simulink model "SM24_model_W"  (R2025b)
settings: Solver=VariableStepAuto  StartTime=0.0  StopTime=T  MaxStep=1e-4  RelTol=1e-3  AbsTol=1e-6
InitFcn:
  | % =========================================================================
  | %  INIT CALLBACK — Simulink Model Workspace
  | %  Sistema de adquisición sísmica SM-24
  | % =========================================================================
  | 
  | %% ========================================================================
  | %  [ SECCIÓN 1: PARÁMETROS CONFIGURABLES ] (Editar solo aquí)
  | %  ========================================================================
  | 
  | % -------------------------------------------------------------------------
  | %  [1.1] Generales
  | % -------------------------------------------------------------------------
  | t_start  = 0;
  | 
  | % -------------------------------------------------------------------------
  | %  [1.2] Geófono SM-24
  | % -------------------------------------------------------------------------
  | fn  = 10;       % Frecuencia natural          (Hz)
  | hi  = 0.25;     % Amortiguamiento interno     (-)
  | G   = 28.8;     % Sensibilidad                (V·s/m)
  | m   = 0.011;    % Masa móvil                  (kg)
  | R_s = 375;      % Resistencia de bobina       (Ohm)
  | 
  | % -------------------------------------------------------------------------
  | %  [1.3] Etapa de Desacople
  | % -------------------------------------------------------------------------
  | R_d  = 1e6;     % Resistencia principal       (Ohm)
  | Ra_d = 10e3;    % Divisora A                  (Ohm)
  | Rb_d = 0;       % Divisora B                  (Ohm)
  | 
  | % -------------------------------------------------------------------------
  | %  [1.4] Diferencial a Single-Ended
  | % -------------------------------------------------------------------------
  | Ra_dse = 10e3;  % (Ohm)
  | Rb_dse = 220e3; % (Ohm)
  | 
  | % -------------------------------------------------------------------------
  | %  [1.5] Etapa de Acondicionamiento (Sallen-Key BP + Sumador)
  | % -------------------------------------------------------------------------
  | R1_bp        = 91000.0;   % (Ohm)
  | Rref_bp      = 82e3;   % (Ohm)
  | Ra_bp        = 22000.0;   % (Ohm)
  | Rb_bp        = 910000.0;  % (Ohm)
  | Rc_bp        = 8200.0;    % (Ohm)
  | C1_bp        = 0.00033;   % (F)
  | C2_bp        = 2.5e-12;   % (F)
  | 
  | Rin_bp_adder = 100000.0+60;  % (Ohm)
  | Rin_u_adder  = 2700.0;    % (Ohm)
  | Rf_add       = 270e3;   % (Ohm)
  | Cf_add       = 1.47e-9;     % (F)
  | Rref_add     = 2.7e3;    % (Ohm)
  | 
  | % -------------------------------------------------------------------------
  | %  [1.6] Filtro Anti-aliasing Analógico
  | % -------------------------------------------------------------------------
  | R1_aa = 270e3;    % (Ohm)
  | R2_aa = 39e3;     % (Ohm)
  | R3_aa = 18e3;     % (Ohm)
  | C1_aa = 33e-9;    % (F)
  | C2_aa = 820e-12;  % (F)
  | 
  | % -------------------------------------------------------------------------
  | %  [1.7] ADC Delta-Sigma
  | % -------------------------------------------------------------------------
  | Decimation_ADC = 64;     % Factor de decimación
  | Fs_ADC         = 3000;   % Frecuencia de muestreo de salida (Hz)
  | Vref           = 2.5;    % (V)
  | 
  | % -------------------------------------------------------------------------
  | %  [1.8] Filtro FIR (Parks-McClellan)
  | % -------------------------------------------------------------------------
  | N_fir = Fs_ADC/2;    % Orden del filtro
  | 
  | % -------------------------------------------------------------------------
  | %  [1.9] Señal de Excitación (3ra Derivada Gaussiana) — Multi-frecuencia
  | % -------------------------------------------------------------------------
  | f_g3_list  = [1];  % Frecuencias de los pulsos (Hz)
  | gap_cycles = 0.5;                          % Ciclos de silencio entre pulsos
  |                                          % (proporcional a cada frecuencia)
  | 
  | % -------------------------------------------------------------------------
  | %  [1.10] Ruido
  | % -------------------------------------------------------------------------
  | nivel_ruido      = 1;    % Ruido gaussiano (amplitud)
  | nivel_ruido_50Hz = 0.2;  % Interferencia de red (amplitud)
  | f_interferencia  = 50;   % Frecuencia de interferencia (Hz)
  | ruido_seed       = 42;   % Semilla fija (reproducibilidad + cache válido)
  | 
  | 
  | %% ========================================================================
  | %  [ SECCIÓN 2: CÁLCULOS Y VARIABLES DERIVADAS ] (No editar)
  | %  ========================================================================
  | 
  | % -------------------------------------------------------------------------
  | %  [2.1] Geófono — parámetros mecánicos y FT
  | % -------------------------------------------------------------------------
  | wn = 2 * pi * fn;
  | k  = m * wn^2;
  | d  = 2 * m * hi * wn;
  | 
  | N_geophone = [0,  wn,       0    ];
  | D_geophone = [1,  2*hi*wn,  wn^2 ];
  | 
  | % -------------------------------------------------------------------------
  | %  [2.2] Tiempos y frecuencias del ADC  (rápido, siempre calcular)
  | % -------------------------------------------------------------------------
  | Ts_ADC = 1 / (Fs_ADC * Decimation_ADC);   % Período modulador (s)
  | Nyq    = Fs_ADC / 2;                       % Frecuencia de Nyquist (Hz)
  | 
  | % -------------------------------------------------------------------------
  | %  [2.3 – 2.5] FIR + Señal + Ruido — con sistema de caché
  | % -------------------------------------------------------------------------
  | 
  | % Parámetros que determinan si el caché es válido
  | cache_file   = 'init_SM24_cache.mat';
  | cache_params = struct( ...
  |     'N_fir',            N_fir,            ...
  |     'Fs_ADC',           Fs_ADC,           ...
  |     'Decimation_ADC',   Decimation_ADC,   ...
  |     'f_g3_list',        f_g3_list,        ...
  |     'gap_cycles',       gap_cycles,       ...
  |     'nivel_ruido',      nivel_ruido,      ...
  |     'nivel_ruido_50Hz', nivel_ruido_50Hz, ...
  |     'f_interferencia',  f_interferencia,  ...
  |     'ruido_seed',       ruido_seed        ...
  | );
  | 
  | cache_valid = false;
  | if isfile(cache_file)
  |     try
  |         cached = load(cache_file);
  |         if isfield(cached, 'cache_params') && isequal(cached.cache_params, cache_params)
  |             cache_valid        = true;
  |             coeficientes_b     = cached.coeficientes_b;
  |             t                  = cached.t;
  |             g3                 = cached.g3;
  |             pulse_info         = cached.pulse_info;
  |             ruido              = cached.ruido;
  |             t_50Hz             = cached.t_50Hz;
  |             ruido_50Hz_diferencial = cached.ruido_50Hz_diferencial;
  |             T                  = cached.T;
  |             t_fir_delay        = cached.t_fir_delay;
  |             fprintf('[CACHE] Cargado desde "%s" — sin cambios detectados.\n', cache_file);
  |         else
  |             fprintf('[CACHE] Parámetros cambiaron — regenerando...\n');
  |         end
  |     catch
  |         fprintf('[CACHE] Archivo inválido — regenerando...\n');
  |     end
  | end
  | 
  | if ~cache_valid
  | 
  |     % -----------------------------------------------------------------------
  |     %  [2.3] Filtro FIR (Parks-McClellan)
  |     % -----------------------------------------------------------------------
  |     fprintf('[FIR] Calculando coeficientes (orden %d) — puede tardar...\n', N_fir);
  |     tic;
  |     coeficientes_b = firpm(N_fir, [0 130, 150 Nyq]/Nyq, [1 1, 0 0], ...
  |                            [1, 1/(10^(-100/20))]);
  |     fprintf('[FIR] Listo en %.1f s\n', toc);
  |     t_fir_delay = (N_fir * 0.75 + 5) / Fs_ADC;   % Latencia del FIR (s)
  | 
  |     % -----------------------------------------------------------------------
  |     %  [2.4] Señal multi-frecuencia (pulsos 3ra derivada gaussiana)
  |     % -----------------------------------------------------------------------
  | 
  |     % Pre-calcular duración de cada pulso y su gap de silencio
  |     sigmas = sqrt(3) ./ (2 * pi * f_g3_list);   % Ancho del pulso
  |     T_g3s  = 10 * sigmas;                        % Duración de cada pulso
  |     gaps   = gap_cycles ./ f_g3_list;            % Silencio proporcional
  | 
  |     % Tiempo total: todos los pulsos + gaps + latencia FIR
  |     T_senal = sum(T_g3s) + sum(gaps) + t_fir_delay;
  |     t       = 0 : Ts_ADC : T_senal;
  |     g3      = zeros(size(t));
  | 
  |     % Tabla de información de cada pulso (útil para análisis posterior)
  |     pulse_info = struct();
  |     pulse_info.freq       = f_g3_list;
  |     pulse_info.t_start    = zeros(size(f_g3_list));
  |     pulse_info.t_end      = zeros(size(f_g3_list));
  |     pulse_info.sigma      = sigmas;
  | 
  |     t_offset = 0;
  |     for k = 1 : numel(f_g3_list)
  |         sigma_k = sigmas(k);
  |         t0_k    = 5 * sigma_k;     % Centro del pulso dentro de su ventana
  |         T_g3_k  = T_g3s(k);
  |         gap_k   = gaps(k);
  | 
  |         t_start_k = t_offset;
  |         t_end_k   = t_offset + T_g3_k;
  | 
  |         % Índices del vector global que pertenecen a este pulso
  |         idx = (t >= t_start_k) & (t < t_end_k);
  | 
  |         % 3ra derivada gaussiana centrada en t0_k dentro de su ventana
  |         tau_k    = t(idx) - (t_start_k + t0_k);
  |         g3_k     = (tau_k .* (tau_k.^2 - 3*sigma_k^2) ./ sigma_k^6) ...
  |                    .* exp(-tau_k.^2 / (2*sigma_k^2));
  | 
  |         % Normalizar cada pulso individualmente a ±0.5
  |         pk = max(abs(g3_k));
  |         if pk > 0
  |             g3(idx) = g3_k / pk * 0.5;
  |         end
  | 
  |         pulse_info.t_start(k) = t_start_k;
  |         pulse_info.t_end(k)   = t_end_k;
  | 
  |         fprintf('[PULSO %d/%d] f=%.1f Hz | t=[%.3f, %.3f] s | sigma=%.4f s\n', ...
  |             k, numel(f_g3_list), f_g3_list(k), t_start_k, t_end_k, sigma_k);
  | 
  |         t_offset = t_end_k + gap_k;
  |     end
  | 
  |     % -----------------------------------------------------------------------
  |     %  [2.5] Generación de ruido (semilla fija para consistencia con caché)
  |     % -----------------------------------------------------------------------
  |     rng(ruido_seed);
  |     ruido = nivel_ruido * randn(size(g3));
  | 
  |     % Interferencia de red — un período completo
  |     t_50Hz                 = 0 : Ts_ADC : (1/f_interferencia - Ts_ADC);
  |     ruido_50Hz_diferencial = nivel_ruido_50Hz * sin(2*pi*f_interferencia*t_50Hz);
  | 
  |     % Duración total de simulación
  |     T = max(t(end), t_50Hz(end));
  | 
  |     % -----------------------------------------------------------------------
  |     %  Guardar caché
  |     % -----------------------------------------------------------------------
  |     save(cache_file, ...
  |         'cache_params', 'coeficientes_b', 't', 'g3', 'pulse_info', ...
  |         'ruido', 't_50Hz', 'ruido_50Hz_diferencial', 'T', 't_fir_delay');
  |     fprintf('[CACHE] Guardado en "%s"\n', cache_file);
  | 
  | end
  | set_param('SM24_model_W/Spectrum Analyzer', ...
  |     'FrequencySpan',  'Start and stop frequencies', ...
  |     'StartFrequency', num2str(min(f_g3_list) / 10), ...
  |     'StopFrequency',  num2str(Nyq));
  | fvtool(coeficientes_b, 1, 'Fs', Fs_ADC);
  | % -----------------------------------------------------------------------
  | %  Resumen final
  | % -----------------------------------------------------------------------
  | fprintf('\n--- Resumen de simulación ---\n');
  | fprintf('  Frecuencias:   %s Hz\n',  mat2str(f_g3_list));
  | fprintf('  T simulación:  %.2f s\n', T);
  | fprintf('  N muestras:    %.2fM\n',  numel(t)/1e6);
  | fprintf('  Ts_ADC:        %.2f µs\n', Ts_ADC*1e6);
  | fprintf('  Latencia FIR:  %.3f s\n', t_fir_delay);
  | fprintf('-----------------------------\n');
values from neighbouring files (symbols this model uses):
  s = tf('s')    [Compensador.m]    (also in compensadorKai.m)
libraries: fl_lib x55, nesl_utility x4, simulink x2, dspmlti4 x1, slctrl_linear x1
CloseFcn:
  | %% Script para unificar datos de Simulink en un solo archivo .mat
  | clear; clc; % <-- BORRAR o dejar comentado si se usa en el StopFcn de Simulink
settings Model: PacingRate=1000  Creator=elias  LastModifiedBy=elias
settings SolverCC: ZeroCrossAlgorithm=Adaptive
settings DebuggingCC: MaskedZcDiagnostic=none  IgnoredZcDiagnostic=none  ParameterPrecisionLossMsg=none
settings RTWCC: GPUComputeCapability=3.5

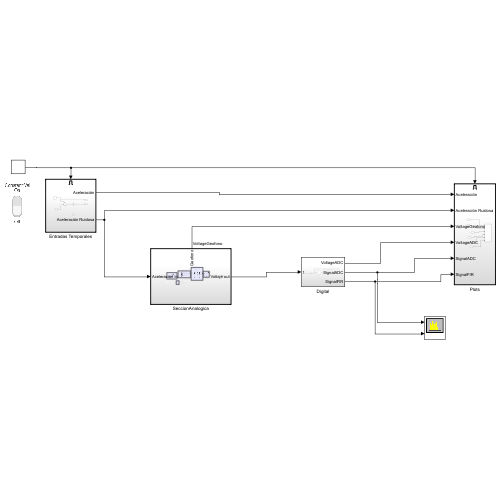
[thumbnail: Simulink's stored preview of the top-level diagram]
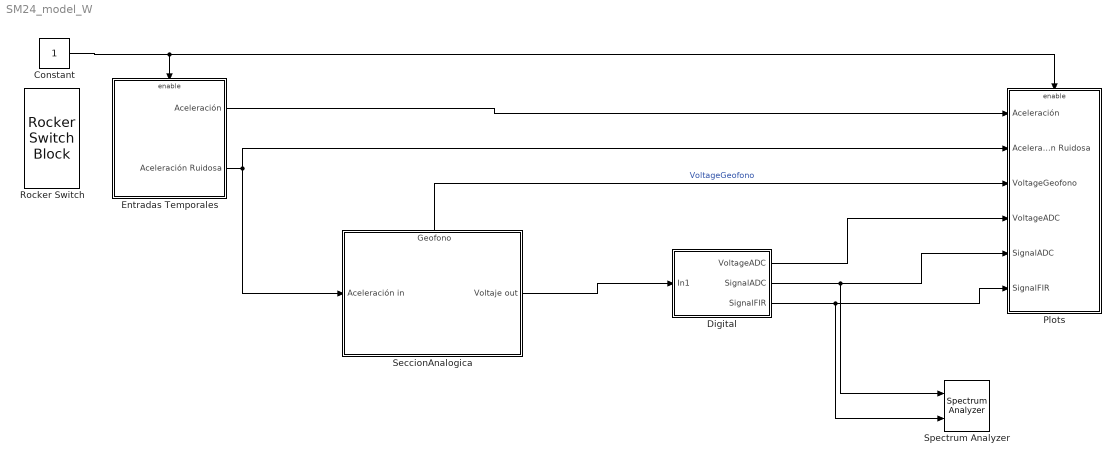
== system SM24_model_W ==
  Constant : Constant
  Digital : Subsystem
  Entradas Temporales : Subsystem
  Plots : Subsystem
  Rocker Switch : RockerSwitchBlock
  SeccionAnalogica : Subsystem  TreatAsAtomicUnit=on
      settings: PortSchema="{\"entries\":[{\"content\":{\"sides\":[{\"content\":{\"connectorIds\":[\"In1\"]},\"type\":\"ConnectorPlacement.EquallySpacedRectSide\",\"uuid\":\"1ba76ad7-8b54-4a44-9f91-ccc3badf3257\"},{\"content\":{\"connectorIds\":[\"Out1\"],\"side\":\"RIGHT\"},\"type\":\"ConnectorPlacement.EquallySpacedRectSide\",\"uuid\":\"9d848629-184e-471f-b904-52491969812c\"},{\"content\":{\"connectorIds\":[\"Out2\"],\"side\":\"TOP\"},\"type\":\"ConnectorPlacement.EquallySpacedRectSide\",\"uuid\":\"a82e2b6d-a8ff-4c30-87e4-e98957da3ec5\"},{\"content\":{\"side\":\"BOTTOM\"},\"type\":\"ConnectorPlacement.EquallySpacedRectSide\",\"uuid\":\"2899f004-1573-4205-9207-50e483759455\"}]},\"type\":\"ConnectorPlacement.EquallySpacedConnector\",\"uuid\":\"1d7f1859-f4c6-4ab5-a8c7-f48e1f148b97\"}],\"packageUris\":[\"http://schema.mathworks.com/mf0/Connector/R2020b\"],\"version\":\"1.0\"}"
  Spectrum Analyzer : SpectrumAnalyzer  NumInputPorts=2  WindowPosition=[481.000000,40.000000,958.000000,1000.000000,]  Visible=on  ScopeFrameLocation=window  ViewType=Spectrum and spectrogram  Method=Welch  SampleRate=44.1e3  PlotAsTwoSidedSpectrum=off  FrequencyScale=Log  WindowInvariantSamplesPerUpdate=on  FrequencySpan=Start and stop frequencies  StartFrequency=0.1  StopFrequency=1500  YLimits=[-3603.4449 -2802.6794]  ColorLimits=[-3603.4449 -2802.6794]  SelectedToolstripTab=spectrumAnalyzerToolstrip.spectrogramTab
  wires:
  SeccionAnalogica/2(Geofono) -> Plots/3(VoltageGeofono)  "VoltageGeofono"
  Constant/1 -> Plots/Enable, Entradas Temporales/Enable
  Entradas Temporales/1(Aceleración) -> Plots/1(Aceleración)
  Digital/3(SignalFIR) -> Spectrum Analyzer/2, Plots/6(SignalFIR)
  SeccionAnalogica/1(Voltaje out) -> Digital/1(In1)
  Digital/1(VoltageADC) -> Plots/4(VoltageADC)
  Digital/2(SignalADC) -> Spectrum Analyzer/1, Plots/5(SignalADC)
  Entradas Temporales/2(Aceleración Ruidosa) -> SeccionAnalogica/1(Aceleración in), Plots/2(Aceleración Ruidosa)

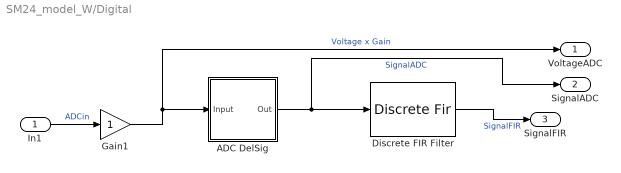
== system SM24_model_W/Digital ==
  In1 : Inport
  ADC DelSig : Subsystem
  Discrete FIR Filter : DiscreteFir  Coefficients=coeficientes_b
  Gain1 : Gain
  VoltageADC : Outport
  SignalADC : Outport  Port=2
  SignalFIR : Outport  Port=3
  wires:
  Discrete FIR Filter/1 -> SignalFIR/1  "SignalFIR"
  Gain1/1 -> VoltageADC/1, ADC DelSig/1(Input)  "Voltage x Gain"
  ADC DelSig/1(Out) -> SignalADC/1, Discrete FIR Filter/1  "SignalADC"
  In1/1 -> Gain1/1  "ADCin"

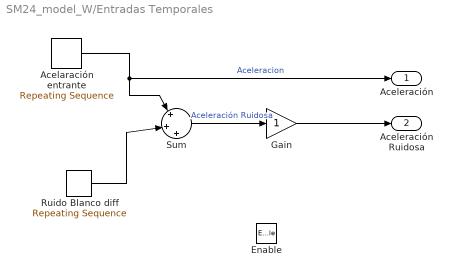
== system SM24_model_W/Entradas Temporales ==
  Enable : EnablePort
  Acelaración entrante : simulink/Sources/Repeating Sequence  rep_seq_t=t  rep_seq_y=g3
  Gain : Gain
  Ruido Blanco diff : simulink/Sources/Repeating Sequence  rep_seq_t=t  rep_seq_y=ruido
  Sum : Sum  Inputs=|+|+|+
  Aceleración : Outport
  Aceleración Ruidosa : Outport  Port=2
  wires:
  Acelaración entrante/1 -> Aceleración/1, Sum/1  "Aceleracion"
  Ruido Blanco diff/1 -> Sum/2
  Sum/1 -> Gain/1  "Aceleración Ruidosa"
  Gain/1 -> Aceleración Ruidosa/1

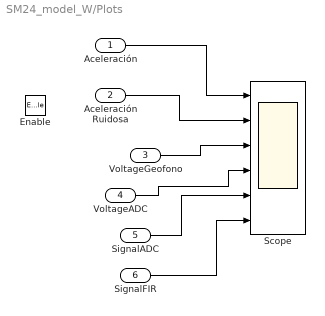
== system SM24_model_W/Plots ==
  Aceleración : Inport
  Aceleración Ruidosa : Inport  Port=2
  VoltageGeofono : Inport  Port=3
  VoltageADC : Inport  Port=4
  SignalADC : Inport  Port=5
  SignalFIR : Inport  Port=6
  Enable : EnablePort
  Scope : Scope  NumInputPorts=6
      settings: ActiveDisplayYMinimum=-89.67264371532174  ActiveDisplayYMaximum=50.94535948326461
  wires:
  Aceleración Ruidosa/1 -> Scope/2
  VoltageADC/1 -> Scope/4
  VoltageGeofono/1 -> Scope/3
  Aceleración/1 -> Scope/1
  SignalFIR/1 -> Scope/6
  SignalADC/1 -> Scope/5

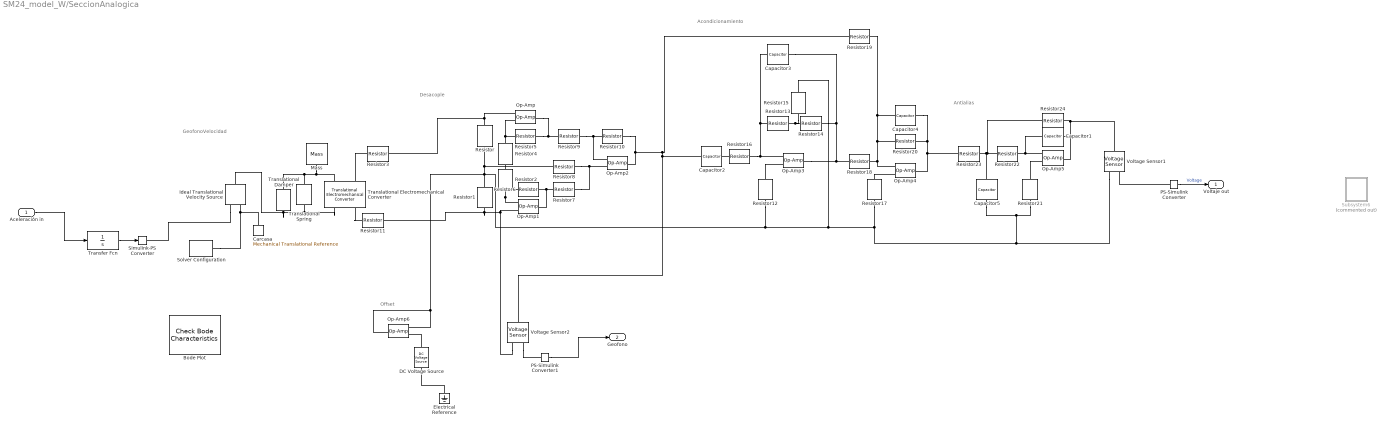
== system SM24_model_W/SeccionAnalogica ==
  note: Antialias
  note: Acondicionamiento
  note: GeofonoVelocidad
  note: Desacople
  note: Offset
  Aceleración in : Inport
  Bode Plot : slctrl_linear/Check Bode  Characteristics  InstantiateOnLoad=on  SaveOperatingPoints=off  LinearizationIOs={'/SeccionAnalogica/PS-Simulink Converter', 1, 'out', 'off', '';'/SeccionAnalogica/PS-Simulink Converter1', 1, 'out', 'off', '';'/SeccionAnalogica/Aceleración in', 1, 'in', 'off', ''}  LinearizeAt=SnapshotTimes  SnapshotTimes=[0]  TriggerType=rising  SampleTime=auto  RateConversionMethod=zoh  PreWarpFreq=10  UseExactDelayModel=off  UseFullBlockNameLabels=off  UseBusSignalLabels=off  enabled=on  stopWhenAssertionFail=off  export=off  ViewDlgPos=[2882 50 958 951]  OpenViewOnLoad=on  LaunchViewOnOpen=on  FrequencyUnits=rad/s  MagnitudeUnits=dB  PhaseUnits=deg  TimeUnits=seconds  EnableUpperBound=off  UpperBoundFrequencies=[]  UpperBoundMagnitudes=[]  EnableLowerBound=off  LowerBoundFrequencies=[]  LowerBoundMagnitudes=[]
      settings: LibrarySourceBlock=slctrlblks/Linear Analysis Plots/Bode Plot  SaveToWorkspace=off  SaveName=sys
  Capacitor1 : fl_lib/Electrical/Electrical Elements/Capacitor  c=C2_aa F  r=0 Ohm  g=0 1/Ohm  i_specify=off  i_priority=None  i=0 A  i_nominal_specify=off  i_nominal_value=1  i_nominal_unit=A  v_specify=off  v_priority=None  v=0 V  v_nominal_specify=off  v_nominal_value=1  v_nominal_unit=V  vc_specify=off  vc_priority=High  vc=0 V  vc_nominal_specify=off  vc_nominal_value=1  vc_nominal_unit=V
  Capacitor2 : fl_lib/Electrical/Electrical Elements/Capacitor  c=C1_bp F  r=0 Ohm  g=0 1/Ohm  i_specify=off  i_priority=None  i=0 A  i_nominal_specify=off  i_nominal_value=1  i_nominal_unit=A  v_specify=off  v_priority=None  v=0 V  v_nominal_specify=off  v_nominal_value=1  v_nominal_unit=V  vc_specify=off  vc_priority=High  vc=0 V  vc_nominal_specify=off  vc_nominal_value=1  vc_nominal_unit=V
  Capacitor3 : fl_lib/Electrical/Electrical Elements/Capacitor  c=C2_bp F  r=0 Ohm  g=0 1/Ohm  i_specify=off  i_priority=None  i=0 A  i_nominal_specify=off  i_nominal_value=1  i_nominal_unit=A  v_specify=off  v_priority=None  v=0 V  v_nominal_specify=off  v_nominal_value=1  v_nominal_unit=V  vc_specify=off  vc_priority=High  vc=0 V  vc_nominal_specify=off  vc_nominal_value=1  vc_nominal_unit=V
  Capacitor4 : fl_lib/Electrical/Electrical Elements/Capacitor  c=Cf_add F  r=0 Ohm  g=0 1/Ohm  i_specify=off  i_priority=None  i=0 A  i_nominal_specify=off  i_nominal_value=1  i_nominal_unit=A  v_specify=off  v_priority=None  v=0 V  v_nominal_specify=off  v_nominal_value=1  v_nominal_unit=V  vc_specify=off  vc_priority=High  vc=0 V  vc_nominal_specify=off  vc_nominal_value=1  vc_nominal_unit=V
  Capacitor5 : fl_lib/Electrical/Electrical Elements/Capacitor  c=C1_aa F  r=0 Ohm  g=0 1/Ohm  i_specify=off  i_priority=None  i=0 A  i_nominal_specify=off  i_nominal_value=1  i_nominal_unit=A  v_specify=off  v_priority=None  v=0 V  v_nominal_specify=off  v_nominal_value=1  v_nominal_unit=V  vc_specify=off  vc_priority=High  vc=0 V  vc_nominal_specify=off  vc_nominal_value=1  vc_nominal_unit=V
  Carcasa : fl_lib/Mechanical/Translational Elements/Mechanical Translational Reference
  DC Voltage Source : fl_lib/Electrical/Electrical Sources/DC Voltage Source  v0=2.5 V
  Electrical Reference : fl_lib/Electrical/Electrical Elements/Electrical Reference
  Ideal Translational Velocity Source : fl_lib/Mechanical/Mechanical Sources/Ideal Translational Velocity Source
  Mass : fl_lib/Mechanical/Translational Elements/Mass  mass=m kg  num_ports=foundation.enum.numPorts2.one  v_specify=off  v_priority=High  v=0 m/s  v_nominal_specify=off  v_nominal_value=1  v_nominal_unit=m/s  f_specify=off  f_priority=None  f=0 N  f_nominal_specify=off  f_nominal_value=1  f_nominal_unit=N
  Op-Amp{,1..6} (7 alike) : fl_lib/Electrical/Electrical Elements/Op-Amp  outI_specify=off  outI_priority=None  outI=0 A  outI_nominal_specify=off  outI_nominal_value=1  outI_nominal_unit=A
  PS-Simulink Converter : nesl_utility/PS-Simulink Converter  PhysicalDomain=network_engine_domain  SubClassName=ps_output  LeftPortType=input  RightPortType=output  PseudoPeriodic=off  Frequencies=[]  VectorFormat=inherit  Unit=inherit  AffineConversion=off
  PS-Simulink Converter1 : nesl_utility/PS-Simulink Converter  PhysicalDomain=network_engine_domain  SubClassName=ps_output  LeftPortType=input  RightPortType=output  PseudoPeriodic=off  Frequencies=[]  VectorFormat=inherit  Unit=inherit  AffineConversion=off
  Resistor : fl_lib/Electrical/Electrical Elements/Resistor  R=R_d Ohm  i_specify=off  i_priority=None  i=0 A  i_nominal_specify=off  i_nominal_value=1  i_nominal_unit=A  v_specify=off  v_priority=None  v=0 V  v_nominal_specify=off  v_nominal_value=1  v_nominal_unit=V
  Resistor1 : fl_lib/Electrical/Electrical Elements/Resistor  R=R_d Ohm  i_specify=off  i_priority=None  i=0 A  i_nominal_specify=off  i_nominal_value=1  i_nominal_unit=A  v_specify=off  v_priority=None  v=0 V  v_nominal_specify=off  v_nominal_value=1  v_nominal_unit=V
  Resistor10 : fl_lib/Electrical/Electrical Elements/Resistor  R=Rb_dse Ohm  i_specify=off  i_priority=None  i=0 A  i_nominal_specify=off  i_nominal_value=1  i_nominal_unit=A  v_specify=off  v_priority=None  v=0 V  v_nominal_specify=off  v_nominal_value=1  v_nominal_unit=V
  Resistor11 : fl_lib/Electrical/Electrical Elements/Resistor  R=R_s/2 Ohm  i_specify=off  i_priority=None  i=0 A  i_nominal_specify=off  i_nominal_value=1  i_nominal_unit=A  v_specify=off  v_priority=None  v=0 V  v_nominal_specify=off  v_nominal_value=1  v_nominal_unit=V
  Resistor12 : fl_lib/Electrical/Electrical Elements/Resistor  R=Rref_bp Ohm  i_specify=off  i_priority=None  i=0 A  i_nominal_specify=off  i_nominal_value=1  i_nominal_unit=A  v_specify=off  v_priority=None  v=0 V  v_nominal_specify=off  v_nominal_value=1  v_nominal_unit=V
  Resistor13 : fl_lib/Electrical/Electrical Elements/Resistor  R=Ra_bp Ohm  i_specify=off  i_priority=None  i=0 A  i_nominal_specify=off  i_nominal_value=1  i_nominal_unit=A  v_specify=off  v_priority=None  v=0 V  v_nominal_specify=off  v_nominal_value=1  v_nominal_unit=V
  Resistor14 : fl_lib/Electrical/Electrical Elements/Resistor  R=Rb_bp Ohm  i_specify=off  i_priority=None  i=0 A  i_nominal_specify=off  i_nominal_value=1  i_nominal_unit=A  v_specify=off  v_priority=None  v=0 V  v_nominal_specify=off  v_nominal_value=1  v_nominal_unit=V
  Resistor15 : fl_lib/Electrical/Electrical Elements/Resistor  R=Rc_bp Ohm  i_specify=off  i_priority=None  i=0 A  i_nominal_specify=off  i_nominal_value=1  i_nominal_unit=A  v_specify=off  v_priority=None  v=0 V  v_nominal_specify=off  v_nominal_value=1  v_nominal_unit=V
  Resistor16 : fl_lib/Electrical/Electrical Elements/Resistor  R=R1_bp Ohm  i_specify=off  i_priority=None  i=0 A  i_nominal_specify=off  i_nominal_value=1  i_nominal_unit=A  v_specify=off  v_priority=None  v=0 V  v_nominal_specify=off  v_nominal_value=1  v_nominal_unit=V
  Resistor17 : fl_lib/Electrical/Electrical Elements/Resistor  R=Rf_add Ohm  i_specify=off  i_priority=None  i=0 A  i_nominal_specify=off  i_nominal_value=1  i_nominal_unit=A  v_specify=off  v_priority=None  v=0 V  v_nominal_specify=off  v_nominal_value=1  v_nominal_unit=V
  Resistor18 : fl_lib/Electrical/Electrical Elements/Resistor  R=Rin_bp_adder Ohm  i_specify=off  i_priority=None  i=0 A  i_nominal_specify=off  i_nominal_value=1  i_nominal_unit=A  v_specify=off  v_priority=None  v=0 V  v_nominal_specify=off  v_nominal_value=1  v_nominal_unit=V
  Resistor19 : fl_lib/Electrical/Electrical Elements/Resistor  R=Rin_u_adder Ohm  i_specify=off  i_priority=None  i=0 A  i_nominal_specify=off  i_nominal_value=1  i_nominal_unit=A  v_specify=off  v_priority=None  v=0 V  v_nominal_specify=off  v_nominal_value=1  v_nominal_unit=V
  Resistor2 : fl_lib/Electrical/Electrical Elements/Resistor  R=Ra_d Ohm  i_specify=off  i_priority=None  i=0 A  i_nominal_specify=off  i_nominal_value=1  i_nominal_unit=A  v_specify=off  v_priority=None  v=0 V  v_nominal_specify=off  v_nominal_value=1  v_nominal_unit=V
  Resistor20 : fl_lib/Electrical/Electrical Elements/Resistor  R=Rf_add Ohm  i_specify=off  i_priority=None  i=0 A  i_nominal_specify=off  i_nominal_value=1  i_nominal_unit=A  v_specify=off  v_priority=None  v=0 V  v_nominal_specify=off  v_nominal_value=1  v_nominal_unit=V
  Resistor21 : fl_lib/Electrical/Electrical Elements/Resistor  R=Rf_add Ohm  i_specify=off  i_priority=None  i=0 A  i_nominal_specify=off  i_nominal_value=1  i_nominal_unit=A  v_specify=off  v_priority=None  v=0 V  v_nominal_specify=off  v_nominal_value=1  v_nominal_unit=V
  Resistor22 : fl_lib/Electrical/Electrical Elements/Resistor  R=R2_aa Ohm  i_specify=off  i_priority=None  i=0 A  i_nominal_specify=off  i_nominal_value=1  i_nominal_unit=A  v_specify=off  v_priority=None  v=0 V  v_nominal_specify=off  v_nominal_value=1  v_nominal_unit=V
  Resistor23 : fl_lib/Electrical/Electrical Elements/Resistor  R=R3_aa Ohm  i_specify=off  i_priority=None  i=0 A  i_nominal_specify=off  i_nominal_value=1  i_nominal_unit=A  v_specify=off  v_priority=None  v=0 V  v_nominal_specify=off  v_nominal_value=1  v_nominal_unit=V
  Resistor24 : fl_lib/Electrical/Electrical Elements/Resistor  R=R1_aa Ohm  i_specify=off  i_priority=None  i=0 A  i_nominal_specify=off  i_nominal_value=1  i_nominal_unit=A  v_specify=off  v_priority=None  v=0 V  v_nominal_specify=off  v_nominal_value=1  v_nominal_unit=V
  Resistor3 : fl_lib/Electrical/Electrical Elements/Resistor  R=R_s/2 Ohm  i_specify=off  i_priority=None  i=0 A  i_nominal_specify=off  i_nominal_value=1  i_nominal_unit=A  v_specify=off  v_priority=None  v=0 V  v_nominal_specify=off  v_nominal_value=1  v_nominal_unit=V
  Resistor4 : fl_lib/Electrical/Electrical Elements/Resistor  R=Ra_d Ohm  i_specify=off  i_priority=None  i=0 A  i_nominal_specify=off  i_nominal_value=1  i_nominal_unit=A  v_specify=off  v_priority=None  v=0 V  v_nominal_specify=off  v_nominal_value=1  v_nominal_unit=V
  Resistor5 : fl_lib/Electrical/Electrical Elements/Resistor  R=Rb_d Ohm  i_specify=off  i_priority=None  i=0 A  i_nominal_specify=off  i_nominal_value=1  i_nominal_unit=A  v_specify=off  v_priority=None  v=0 V  v_nominal_specify=off  v_nominal_value=1  v_nominal_unit=V
  Resistor6 : fl_lib/Electrical/Electrical Elements/Resistor  R=Rb_d Ohm  i_specify=off  i_priority=None  i=0 A  i_nominal_specify=off  i_nominal_value=1  i_nominal_unit=A  v_specify=off  v_priority=None  v=0 V  v_nominal_specify=off  v_nominal_value=1  v_nominal_unit=V
  Resistor7 : fl_lib/Electrical/Electrical Elements/Resistor  R=Ra_dse Ohm  i_specify=off  i_priority=None  i=0 A  i_nominal_specify=off  i_nominal_value=1  i_nominal_unit=A  v_specify=off  v_priority=None  v=0 V  v_nominal_specify=off  v_nominal_value=1  v_nominal_unit=V
  Resistor8 : fl_lib/Electrical/Electrical Elements/Resistor  R=Rb_dse Ohm  i_specify=off  i_priority=None  i=0 A  i_nominal_specify=off  i_nominal_value=1  i_nominal_unit=A  v_specify=off  v_priority=None  v=0 V  v_nominal_specify=off  v_nominal_value=1  v_nominal_unit=V
  Resistor9 : fl_lib/Electrical/Electrical Elements/Resistor  R=Ra_dse Ohm  i_specify=off  i_priority=None  i=0 A  i_nominal_specify=off  i_nominal_value=1  i_nominal_unit=A  v_specify=off  v_priority=None  v=0 V  v_nominal_specify=off  v_nominal_value=1  v_nominal_unit=V
  Simulink-PS Converter : nesl_utility/Simulink-PS Converter  PhysicalDomain=network_engine_domain  SubClassName=ps_input  LeftPortType=input  RightPortType=output  PseudoPeriodic=off  Frequencies=[]  NoiseDistribution=none  NoiseParameters=[]  Unit=1  AffineConversion=off  FilteringAndDerivatives=provide  SimscapeFilterOrder=1  InputFilterTimeConstant=0.001  UdotUserProvided=0
  Solver Configuration : nesl_utility/Solver Configuration  PhysicalDomain=network_engine_domain  SubClassName=solver  LeftPortType=input  RightPortType=generic  Tones=[]  Harmonics=[]  SimulateNoise=off  Profile=off  UseLocalSampling=off  EnableSwitchedLinearOptims=on  FrequencyDomain=off  UseCCode=off  RelTol=0.001  AbsTol=0.001  MinStep=1e-09  ToWorkspace=off  RevertToSquareIcSolve=off  NumHomotopyIterations=100  PhasorMode=off  PhasorModeNumHarmonics=1  ConsistencySolver=NEWTON_XTOL_AFTER_FTOL  IndexReductionMethod=DerivativeReplacement  DoDC=on  ResidualTolerance=1e-09  ConsistencyTolSource=GLOBAL  ConsistencyAbsTol=0.001  ConsistencyRelTol=0.001  ConsistencyTolFactor=0.001  UseLocalSolver=off  LocalSolverChoice=NE_BACKWARD_EULER_ADVANCER  ResolveIndetEquations=on  FunctionEvalNumThread=1  LocalSolverSampleTime=0.001  DoFixedCost=off  MaxNonlinIter=3  MaxModeIter=2  ComputeImpulses=off  ImpulseIterations=2  LinearAlgebra=auto  LinearAlgebraNumThread=0  EquationFormulation=NE_TIME_EF  DelaysMemoryBudget=1024  AutomaticFiltering=off  FilteringTimeConstant=0.001  PartitionStorageMethod=AS_NEEDED  PartitionMemoryBudget=1024  PartitionMethod=ROBUST  MultibodyUseLocalSolver=off  MultibodyLocalSolverChoice=ODE1  MultibodyLocalSolverSampleTime=0.001
  Subsystem6 : Subsystem  Commented=on
  Transfer Fcn : TransferFcn  Denominator=[1 0]
  Translational Electromechanical Converter : fl_lib/Electrical/Electrical Elements/Translational Electromechanical Converter  K=G V*s/m  i_specify=off  i_priority=None  i=0 A  i_nominal_specify=off  i_nominal_value=1  i_nominal_unit=A  v_specify=off  v_priority=None  v=0 V  v_nominal_specify=on  v_nominal_value=1  v_nominal_unit=V  f_specify=off  f_priority=None  f=0 N  f_nominal_specify=off  f_nominal_value=1  f_nominal_unit=N  u_specify=off  u_priority=None  u=0 m/s  u_nominal_specify=on  u_nominal_value=1  u_nominal_unit=m/s
      settings: InternalSimscapePortConfiguration="{\"Bottom\":[],\"Left\":[{\"id\":\"p\",\"label\":\"+\",\"type\":\"foundation.electrical.electrical\"},{\"id\":\"R\",\"label\":\"R\",\"type\":\"foundation.mechanical.translational.translational\"}],\"Right\":[{\"id\":\"n\",\"label\":\"-\",\"type\":\"foundation.electrical.electrical\"},{\"id\":\"C\",\"label\":\"C\",\"type\":\"foundation.mechanical.translational.translational\"}],\"Top\":[]}"
  Translational Damper : fl_lib/Mechanical/Translational Elements/Translational Damper  D=d N*s/m  v_specify=off  v_priority=None  v=0 m/s  v_nominal_specify=off  v_nominal_value=1  v_nominal_unit=m/s  f_specify=off  f_priority=None  f=0 N  f_nominal_specify=off  f_nominal_value=1  f_nominal_unit=N
  Translational Spring : fl_lib/Mechanical/Translational Elements/Translational Spring  spr_rate=k N/m  v_specify=off  v_priority=None  v=0 m/s  v_nominal_specify=off  v_nominal_value=1  v_nominal_unit=m/s  f_specify=off  f_priority=None  f=0 N  f_nominal_specify=off  f_nominal_value=1  f_nominal_unit=N  x_specify=off  x_priority=High  x=0 m  x_nominal_specify=off  x_nominal_value=1  x_nominal_unit=m
  Voltage Sensor1 : fl_lib/Electrical/Electrical Sensors/Voltage Sensor
  Voltage Sensor2 : fl_lib/Electrical/Electrical Sensors/Voltage Sensor
  Voltaje out : Outport
  Geofono : Outport  Port=2
  wires:
  PS-Simulink Converter1/1 -> Geofono/1
  Transfer Fcn/1 -> Simulink-PS Converter/1
  PS-Simulink Converter/1 -> Voltaje out/1  "Voltage"
  Aceleración in/1 -> Transfer Fcn/1
  connections:
  PS-Simulink Converter/LConn1 -- Voltage Sensor1/RConn1
  Resistor1/RConn1 -- Resistor15/RConn1 -- Capacitor5/RConn1 -- Resistor21/RConn1 -- Voltage Sensor1/RConn2 -- Resistor17/RConn1 -- Resistor12/RConn1 -- Op-Amp6/LConn1 -- Op-Amp6/RConn1 -- Resistor8/LConn1 -- Resistor/LConn1
  Ideal Translational Velocity Source/RConn1 -- Simulink-PS Converter/RConn1
  Resistor2/LConn1 -- Op-Amp1/LConn2 -- Resistor6/LConn1
  Electrical Reference/LConn1 -- DC Voltage Source/RConn1
  Resistor6/RConn1 -- Op-Amp1/RConn1 -- Resistor7/LConn1
  Translational Electromechanical Converter/LConn1 -- Resistor3/LConn1
  Resistor5/RConn1 -- Op-Amp/RConn1 -- Resistor9/LConn1
  Translational Damper/RConn1 -- Ideal Translational Velocity Source/LConn1 -- Translational Electromechanical Converter/RConn2 -- Translational Spring/RConn1
  Resistor4/RConn1 -- Op-Amp/LConn2 -- Resistor5/LConn1
  Translational Spring/LConn1 -- Translational Electromechanical Converter/LConn2 -- Mass/LConn1 -- Translational Damper/LConn1
  DC Voltage Source/LConn1 -- Op-Amp6/LConn2
  Carcasa/LConn1 -- Solver Configuration/RConn1 -- Ideal Translational Velocity Source/RConn2
  Resistor1/LConn1 -- Op-Amp1/LConn1 -- Voltage Sensor2/RConn2 -- Resistor11/RConn1
  Voltage Sensor2/RConn1 -- PS-Simulink Converter1/LConn1
  Resistor7/RConn1 -- Op-Amp2/LConn1 -- Resistor8/RConn1
  Resistor9/RConn1 -- Resistor10/LConn1 -- Op-Amp2/LConn2
  Resistor2/RConn1 -- Resistor4/LConn1
  Resistor11/LConn1 -- Translational Electromechanical Converter/RConn1
  Resistor/RConn1 -- Op-Amp/LConn1 -- Resistor3/RConn1
  Resistor12/LConn1 -- Op-Amp3/LConn1
  Capacitor3/LConn1 -- Op-Amp3/LConn2 -- Resistor16/LConn1 -- Resistor13/RConn1
  Resistor10/RConn1 -- Voltage Sensor2/LConn1 -- Capacitor2/LConn1 -- Resistor19/LConn1 -- Op-Amp2/RConn1
  Op-Amp4/LConn1 -- Resistor17/LConn1
  Resistor18/RConn1 -- Op-Amp4/LConn2 -- Resistor19/RConn1 -- Capacitor4/LConn1 -- Resistor20/LConn1
  Capacitor4/RConn1 -- Resistor23/LConn1 -- Op-Amp4/RConn1 -- Resistor20/RConn1
  Resistor21/LConn1 -- Op-Amp5/LConn1
  Resistor22/RConn1 -- Op-Amp5/LConn2 -- Capacitor1/LConn1
  Capacitor1/RConn1 -- Voltage Sensor1/LConn1 -- Resistor24/RConn1 -- Op-Amp5/RConn1
  Resistor23/RConn1 -- Resistor22/LConn1 -- Resistor24/LConn1 -- Capacitor5/LConn1
  Resistor18/LConn1 -- Capacitor3/RConn1 -- Resistor14/LConn1 -- Op-Amp3/RConn1
  Capacitor2/RConn1 -- Resistor16/RConn1
  Resistor15/LConn1 -- Resistor13/LConn1 -- Resistor14/RConn1

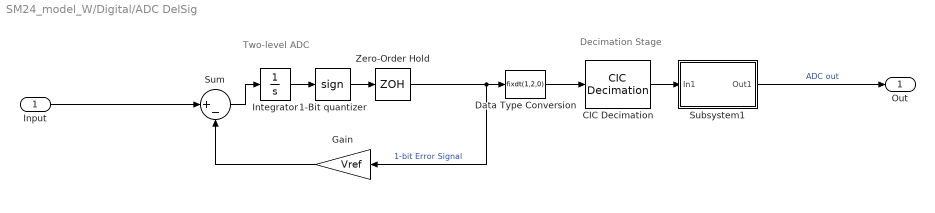
== system SM24_model_W/Digital/ADC DelSig ==
  note: Two-level ADC
  note: Decimation Stage
  Input : Inport
  1-Bit quantizer : Signum
  CIC Decimation : dspmlti4/CIC Decimation  filtFrom=Dialog parameters  filtobj=Hm_decim  ftype=Decimator  R=Decimation_ADC  M=1  N=5  filterInternals=Full precision  BPS=[32 30 24 20 16 16 16 16 16 16]  FLPS=0  outputWordLength=16  outputFracLength=0  launchFVT=off  framing=Maintain input frame rate  RateOptions=Allow multirate processing
  Data Type Conversion : DataTypeConversion  OutDataTypeStr=fixdt(1,2,0)  SaturateOnIntegerOverflow=off  RndMeth=Floor
  Gain : Gain  Gain=Vref
  Integrator : Integrator
  Subsystem1 : Subsystem
      mask Display: disp('Rescaling for\nComparison')
  Sum : Sum  Inputs=|+-  InputSameDT=on  SaturateOnIntegerOverflow=on  OutDataTypeStr=Inherit: Same as first input
  Zero-Order Hold : ZeroOrderHold  SampleTime=Ts_ADC
  Out : Outport
  wires:
  Data Type Conversion/1 -> CIC Decimation/1
  Zero-Order Hold/1 -> Gain/1, Data Type Conversion/1  "1-bit Error Signal"
  Integrator/1 -> 1-Bit quantizer/1
  1-Bit quantizer/1 -> Zero-Order Hold/1
  Sum/1 -> Integrator/1
  Input/1 -> Sum/1
  CIC Decimation/1 -> Subsystem1/1(In1)
  Subsystem1/1(Out1) -> Out/1  "ADC out"
  Gain/1 -> Sum/2

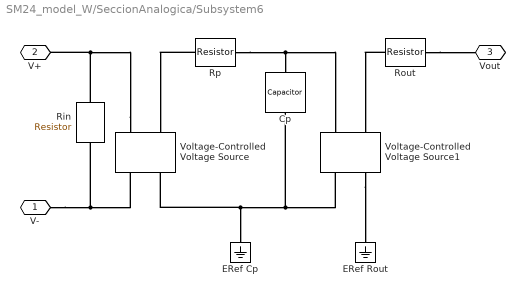
== system SM24_model_W/SeccionAnalogica/Subsystem6 ==
  Cp : fl_lib/Electrical/Electrical Elements/Capacitor  Tag=Factory Generic  c=1/(2*pi*8e6*100) F  r=0 Ohm  g=0 1/Ohm  i_specify=off  i_priority=High  i=0 A  i_nominal_specify=off  i_nominal_value=1  i_nominal_unit=A  v_specify=off  v_priority=High  v=0 V  v_nominal_specify=off  v_nominal_value=1  v_nominal_unit=V  vc_specify=on  vc_priority=High  vc=0 V  vc_nominal_specify=off  vc_nominal_value=1  vc_nominal_unit=V
  ERef Cp : fl_lib/Electrical/Electrical Elements/Electrical Reference  Tag=Factory Generic
  ERef Rout : fl_lib/Electrical/Electrical Elements/Electrical Reference  Tag=Factory Generic
  Rin : fl_lib/Electrical/Electrical Elements/Resistor  Tag=Factory Generic  R=35e6 Ohm  i_specify=off  i_priority=High  i=0 A  i_nominal_specify=off  i_nominal_value=1  i_nominal_unit=A  v_specify=off  v_priority=High  v=0 V  v_nominal_specify=off  v_nominal_value=1  v_nominal_unit=V
  Rout : fl_lib/Electrical/Electrical Elements/Resistor  Tag=Factory Generic  R=20 Ohm  i_specify=off  i_priority=High  i=0 A  i_nominal_specify=off  i_nominal_value=1  i_nominal_unit=A  v_specify=off  v_priority=High  v=0 V  v_nominal_specify=off  v_nominal_value=1  v_nominal_unit=V
  Rp : fl_lib/Electrical/Electrical Elements/Resistor  Tag=Factory Generic  R=100 Ohm  i_specify=off  i_priority=High  i=0 A  i_nominal_specify=off  i_nominal_value=1  i_nominal_unit=A  v_specify=off  v_priority=High  v=0 V  v_nominal_specify=off  v_nominal_value=1  v_nominal_unit=V
  Voltage-Controlled Voltage Source : fl_lib/Electrical/Electrical Sources/Voltage-Controlled Voltage Source  K=sqrt(10)*10e3  v1_specify=off  v1_priority=High  v1=0 V  v1_nominal_specify=off  v1_nominal_value=1  v1_nominal_unit=V  v2_specify=off  v2_priority=High  v2=0 V  v2_nominal_specify=off  v2_nominal_value=1  v2_nominal_unit=V
      settings: InternalSimscapePortConfiguration="{\"Bottom\":[],\"Left\":[{\"id\":\"p1\",\"label\":\"+\",\"type\":\"foundation.electrical.electrical\"},{\"id\":\"p2\",\"label\":\"+\",\"type\":\"foundation.electrical.electrical\"}],\"Right\":[{\"id\":\"n1\",\"label\":\"-\",\"type\":\"foundation.electrical.electrical\"},{\"id\":\"n2\",\"label\":\"-\",\"type\":\"foundation.electrical.electrical\"}],\"Top\":[]}"
  Voltage-Controlled Voltage Source1 : fl_lib/Electrical/Electrical Sources/Voltage-Controlled Voltage Source  K=1  v1_specify=off  v1_priority=High  v1=0 V  v1_nominal_specify=off  v1_nominal_value=1  v1_nominal_unit=V  v2_specify=off  v2_priority=High  v2=0 V  v2_nominal_specify=off  v2_nominal_value=1  v2_nominal_unit=V
      settings: InternalSimscapePortConfiguration="{\"Bottom\":[],\"Left\":[{\"id\":\"p1\",\"label\":\"+\",\"type\":\"foundation.electrical.electrical\"},{\"id\":\"p2\",\"label\":\"+\",\"type\":\"foundation.electrical.electrical\"}],\"Right\":[{\"id\":\"n1\",\"label\":\"-\",\"type\":\"foundation.electrical.electrical\"},{\"id\":\"n2\",\"label\":\"-\",\"type\":\"foundation.electrical.electrical\"}],\"Top\":[]}"
  V- : PMIOPort  Side=Left
  V+ : PMIOPort  Port=2  Side=Left
  Vout : PMIOPort  Port=3  Side=Right
  connections:
  Rout/RConn1 -- Voltage-Controlled Voltage Source1/LConn2
  Voltage-Controlled Voltage Source1/RConn2 -- ERef Rout/LConn1
  Voltage-Controlled Voltage Source/RConn1 -- Rin/RConn1 -- V-/RConn1
  Voltage-Controlled Voltage Source1/RConn1 -- Cp/RConn1 -- ERef Cp/LConn1 -- Voltage-Controlled Voltage Source/RConn2
  Rp/LConn1 -- Cp/LConn1 -- Voltage-Controlled Voltage Source1/LConn1
  Rout/LConn1 -- Vout/RConn1
  Voltage-Controlled Voltage Source/LConn1 -- Rin/LConn1 -- V+/RConn1
  Rp/RConn1 -- Voltage-Controlled Voltage Source/LConn2

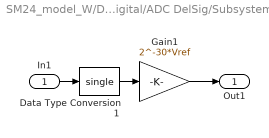
== system SM24_model_W/Digital/ADC DelSig/Subsystem1 ==
  In1 : Inport
  Data Type Conversion1 : DataTypeConversion  OutDataTypeStr=single  SaturateOnIntegerOverflow=off  RndMeth=Floor
  Gain1 : Gain  Gain=2^-30*Vref  SaturateOnIntegerOverflow=on  OutDataTypeStr=Inherit: Same as input  ParamDataTypeStr=Inherit: Same as input
  Out1 : Outport  VectorParamsAs1DForOutWhenUnconnected=off
  wires:
  Data Type Conversion1/1 -> Gain1/1
  In1/1 -> Data Type Conversion1/1
  Gain1/1 -> Out1/1
